simulink model "SMC_20231127"  (R2021b)
settings: Solver=VariableStepAuto  StartTime=0.0  StopTime=40  RelTol=1e-3
settings Model: Creator=旧友  LastModifiedBy=旧友

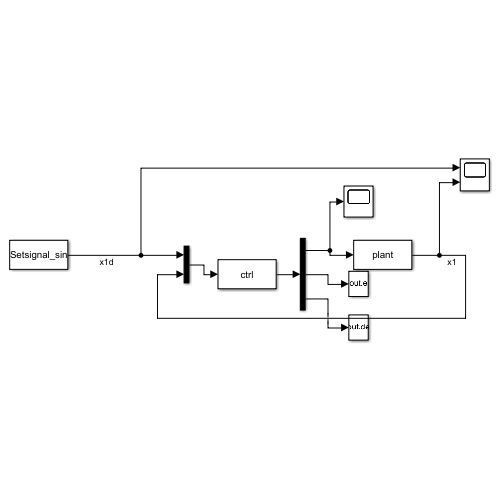
[thumbnail: Simulink's stored preview of the top-level diagram]
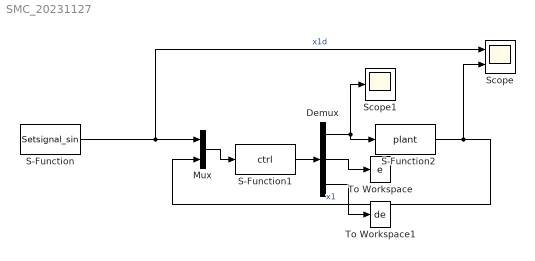
== system SMC_20231127 ==
  Demux : Demux  Outputs=3
  Mux : Mux  Inputs=2
  S-Function : S-Function  FunctionName=Setsignal_sin  Parameters=pa  SFunctionDeploymentMode=off  EnableBusSupport=off
  S-Function1 : S-Function  FunctionName=ctrl  Parameters=pa  SFunctionDeploymentMode=off  EnableBusSupport=off
  S-Function2 : S-Function  FunctionName=plant  Parameters=pa  SFunctionDeploymentMode=off  EnableBusSupport=off
  Scope : Scope  NumInputPorts=2
  Scope1 : Scope
  To Workspace : ToWorkspace  VariableName=e  SampleTime=-1
  To Workspace1 : ToWorkspace  VariableName=de  SampleTime=-1
  wires:
  S-Function/1 -> Scope/1, Mux/1  "x1d"
  S-Function2/1 -> Scope/2, Mux/2  "x1"
  Mux/1 -> S-Function1/1
  S-Function1/1 -> Demux/1
  Demux/1 -> Scope1/1, S-Function2/1
  Demux/2 -> To Workspace/1
  Demux/3 -> To Workspace1/1
